simulink model "SCR_FW"  (R2019a)
settings: Solver=ode23  StartTime=0.0  StopTime=0.05  RelTol=1e-3
libraries: powerlib x12
settings Model: Creator=Amanna  LastModifiedBy=Amanna
settings DataIOCC: ReturnWorkspaceOutputs=off

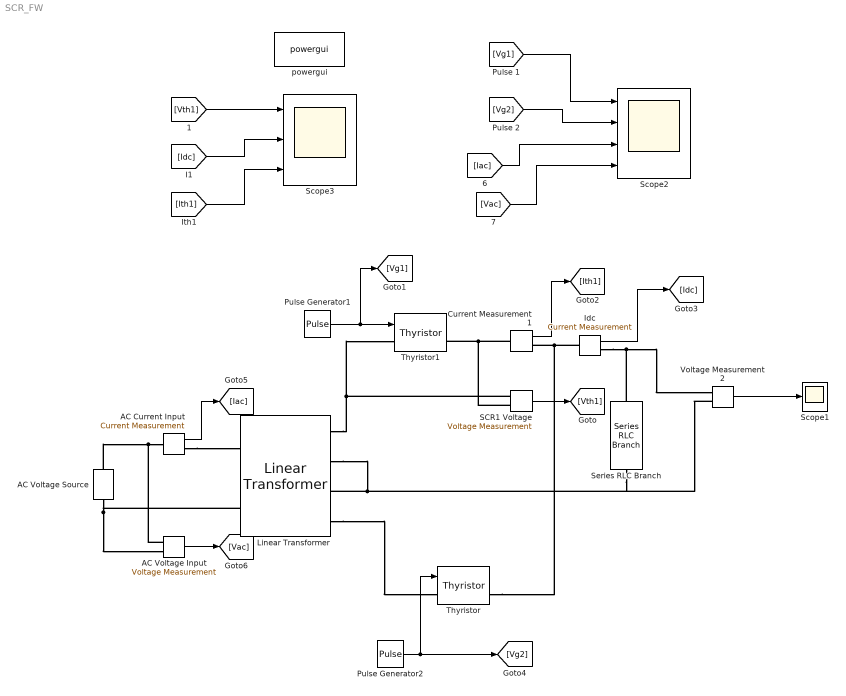
== system SCR_FW ==
  AC Current Input : powerlib/Measurements/Current Measurement  PhasorSimulation=off  OutputType=Complex  PSBequivalent=0
      settings: SourceProductName=Simscape Electrical
  AC Voltage Input : powerlib/Measurements/Voltage Measurement  PhasorSimulation=off  OutputType=Complex  PSBequivalent=0
      settings: SourceProductName=Simscape Electrical
  AC Voltage Source : powerlib/Electrical Sources/AC Voltage Source  Amplitude=230  Phase=0  Frequency=50  SampleTime=0  Measurements=None  BusType=swing  Pref=10e3  Qref=0  Qmin=-inf  Qmax=+inf
      settings: SourceProductName=Simscape Electrical
  Current Measurement1 : powerlib/Measurements/Current Measurement  PhasorSimulation=off  OutputType=Complex  PSBequivalent=0
      settings: SourceProductName=Simscape Electrical
  Idc : powerlib/Measurements/Current Measurement  PhasorSimulation=off  OutputType=Complex  PSBequivalent=0
      settings: SourceProductName=Simscape Electrical
  Linear Transformer : powerlib/Elements/Linear Transformer  UNITS=SI  NominalPower=[ 250e3 50 ]  winding1=[400*0.707 4.3218 0]  winding2=[200*0.707 0.7938 0]  ThreeWindings=on  winding3=[200*0.707 0.7938 0]  RmLm=[1.0805e+06 2866]  Measurements=None  DataType=on
      settings: SourceProductName=Simscape Electrical
  Pulse Generator1 : DiscretePulseGenerator  PulseType=Time based  Amplitude=50  Period=0.02  PulseWidth=20  PhaseDelay=1.667e-3
  Pulse Generator2 : DiscretePulseGenerator  PulseType=Time based  Amplitude=50  Period=0.02  PulseWidth=20  PhaseDelay=0.011667
  SCR1 Voltage : powerlib/Measurements/Voltage Measurement  PhasorSimulation=off  OutputType=Complex  PSBequivalent=0
      settings: SourceProductName=Simscape Electrical
  Scope1 : Scope
  Scope2 : Scope  NumInputPorts=4
  Scope3 : Scope  NumInputPorts=3
  Series RLC Branch : powerlib/Elements/Series RLC Branch  LConnTagsString=__new0  RConnTagsString=__new0  BranchType=R  Resistance=1  Inductance=1e-3  SetiL0=off  InitialCurrent=0  Capacitance=1e-6  Setx0=off  InitialVoltage=0  Measurements=None
      settings: SourceProductName=Simscape Electrical
  Thyristor : powerlib/Power Electronics/Thyristor  Ron=0.001  Lon=0  Vf=0.8  IC=0  Rs=500  Cs=250e-9  Measurements=on
      settings: SourceProductName=Simscape Electrical
  Thyristor1 : powerlib/Power Electronics/Thyristor  Ron=0.001  Lon=0  Vf=0.8  IC=0  Rs=500  Cs=250e-9  Measurements=on
      settings: SourceProductName=Simscape Electrical
  Voltage Measurement2 : powerlib/Measurements/Voltage Measurement  PhasorSimulation=off  OutputType=Complex  PSBequivalent=0
      settings: SourceProductName=Simscape Electrical
  powergui : powerlib/powergui  Priority=1  SimulationMode=Continuous  SampleTime=50e-6  frequency=60  Iterations=50  frequencyindice=50  Pbase=100e6  ErrMax=1e-4  UnitsV=kV  UnitsW=MW  buscounter=0  FunctionMessages=off  echomessages=off  EnableUseOfTLC=off  CurrentSourceSwitches=off  DisableSnubberDevices=on  DisableRonSwitches=on  DisableVfSwitches=off  DisplayEquations=off  AutomaticDiscreteSolvers=off  SolverType=Tustin/Backward Euler (TBE)  Interpol=off  ExternalGateDelay=off  methode=off  Ts=100  x0status=blocks  SPID=on  SwTol=0  HookPort=off  NonlinearTolerance=0  nMaxIteration=15  ContinueOnMaxIteration=off  RestoreLinks=warning  ResistiveCurrentMeasurement=off  Frange=[0:2:500]  Ylog=off  Xlog=on  ShowGrid=off  save=off  variable=ZData  structure=Signals1  ZoomFFT=off  StartTime=0.02  cycles=1  DisplayStyle=1  fundamental=50  FreqAxis=off  MaxFrequency=1000  frequencyindicesteady=1  RmsSteady=1  display=off
      settings: SourceProductName=Simscape Electrical
  wires:
  Pulse Generator1/1 -> [Vg1], Thyristor1/1
  Pulse Generator2/1 -> [Vg2], Thyristor/1
  SCR1 Voltage/1 -> [Vth1]
  Current Measurement1/1 -> [Ith1]
  Idc/1 -> [Idc]
  Voltage Measurement2/1 -> Scope1/1
  AC Current Input/1 -> [Iac]
  AC Voltage Input/1 -> [Vac]
  [Vg1] -> Scope2/1
  [Vg2] -> Scope2/2
  [Iac] -> Scope2/3
  [Vac] -> Scope2/4
  [Idc] -> Scope3/2
  [Vth1] -> Scope3/1
  [Ith1] -> Scope3/3
  connections:
  Linear Transformer/RConn1 -- Thyristor1/LConn1 -- SCR1 Voltage/LConn1
  Linear Transformer/RConn2 -- Series RLC Branch/RConn1 -- Voltage Measurement2/LConn2 -- Linear Transformer/RConn3
  Linear Transformer/RConn4 -- Thyristor/LConn1
  Current Measurement1/LConn1 -- SCR1 Voltage/LConn2 -- Thyristor1/RConn1
  AC Current Input/RConn1 -- Linear Transformer/LConn1
  AC Voltage Source/RConn1 -- AC Voltage Input/LConn1 -- AC Current Input/LConn1
  AC Voltage Source/LConn1 -- AC Voltage Input/LConn2 -- Linear Transformer/LConn2
  Idc/LConn1 -- Thyristor/RConn1 -- Current Measurement1/RConn1
  Idc/RConn1 -- Series RLC Branch/LConn1 -- Voltage Measurement2/LConn1
